simulink model "Task_No4"  (R2023b)
settings: Solver=ode5  StartTime=0.0  StopTime=3600*24*7  FixedStep=1  RelTol=1e-3
InitFcn:
  | PARAMETERS;
StartFcn:
  | PARAMETERS;
values from neighbouring files (symbols this model uses):
  Conv_C_to_K = 273.15    [PARAMETERS.m]
  P_AREA_WALL = sqrt(P_AREA_BDR)*P_RM_HEIGHT-P_AREA_WIN    [PARAMETERS.m]
  P_AREA_WIN = 1.82    [PARAMETERS.m]
  P_CP_AIR = 1012    [PARAMETERS.m]
  P_EM_GLASS = 0.94    [PARAMETERS.m]
  P_EM_WALL = 0.94    [PARAMETERS.m]
  P_HEATER_AIR_FLOW = 1    [PARAMETERS.m]
  R_WALL = 1/(U_WALL*P_AREA_WALL)    [PARAMETERS.m]
  R_WINDOW = 1/(U_WINDOW*P_AREA_WIN)    (= 0.18315018315)    [PARAMETERS.m]
  T_HEATER = 50    [PARAMETERS.m]
  T_INIT_BDR = 18    [PARAMETERS.m]
  T_INIT_OUT = 2.9    [PARAMETERS.m]
undefined symbols (not defined in the file or in its folder): TBL_TEMP
libraries: fl_lib x21, nesl_utility x8, slpidlib x1
settings Model: Creator=Selim  LastModifiedBy=Selim

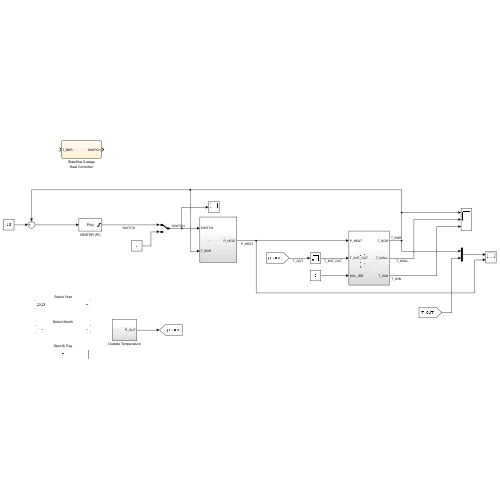
[thumbnail: Simulink's stored preview of the top-level diagram]
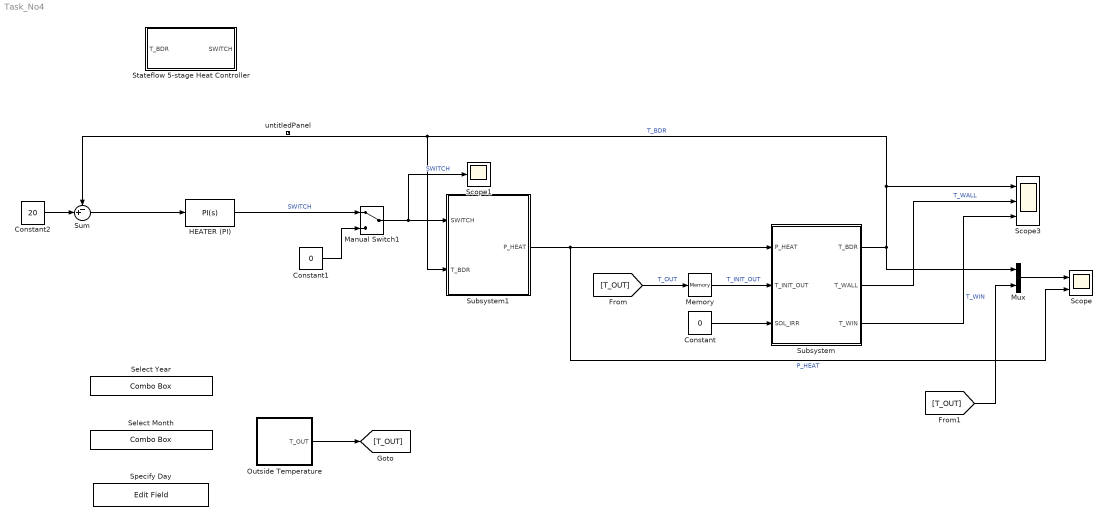
== system Task_No4 ==
  Constant : Constant  Value=0
  Constant1 : Constant  Value=0
  Constant2 : Constant  Value=20
  HEATER (PI) : slpidlib/PID Controller  Controller=PI  Form=Parallel  TimeDomain=Continuous-time  UseExternalTs=off  SampleTime=-1  IntegratorMethod=Forward Euler  FilterMethod=Forward Euler  ControllerParametersSource=internal  P=0.143081964564318  I=0.00336579194559755  UseKiTs=off  D=39.5738922859411  N=3204.37920267902  UseFilter=on  TunerSelectOption=Transfer Function Based (PID Tuner App)  InitialConditionSource=internal  InitialConditionForIntegrator=0  InitialConditionForFilter=0  DifferentiatorICPrevScaledInput=0  ExternalReset=none  TrackingMode=off  Kt=1  LimitOutput=on  SatLimitsSource=internal  UpperSaturationLimit=1  LowerSaturationLimit=0  LinearizeAsGain=on  AntiWindupMode=clamping  Kb=1  LimitIntegrator=off  UpperIntegratorSaturationLimit=inf  LowerIntegratorSaturationLimit=-inf  POutMin=[]  POutMax=[]  IOutMin=[]  IOutMax=[]  DOutMin=[]  DOutMax=[]  NOutMin=[]  NOutMax=[]  SumOutMin=[]  SumOutMax=[]  SaturationOutMin=[]  SaturationOutMax=[]  PParamMin=[]  PParamMax=[]  IParamMin=[]  IParamMax=[]  DParamMin=[]  DParamMax=[]  NParamMin=[]  NParamMax=[]  KbParamMin=[]  KbParamMax=[]  KtParamMin=[]  KtParamMax=[]  KbOutMin=[]  KbOutMax=[]  KtOutMin=[]  KtOutMax=[]  IntegratorOutMin=[]  IntegratorOutMax=[]  FilterOutMin=[]  FilterOutMax=[]  SumI1OutMin=[]  SumI1OutMax=[]  SumI2OutMin=[]  SumI2OutMax=[]  SumI3OutMin=[]  SumI3OutMax=[]  SumI4OutMin=[]  SumI4OutMax=[]  SumDOutMin=[]  SumDOutMax=[]  DifferentiatorOutMin=[]  DifferentiatorOutMax=[]  FilterDiffOutCoefMin=[]  FilterDiffOutCoefMax=[]  ReciprocalOutMin=[]  ReciprocalOutMax=[]  SumDenOutMin=[]  SumDenOutMax=[]  SumNumOutMin=[]  SumNumOutMax=[]  DivideOutMin=[]  DivideOutMax=[]  UdiffTsProdOutMin=[]  UdiffTsProdOutMax=[]  NTsProdOutMin=[]  NTsProdOutMax=[]  UintegralTsProdOutMin=[]  UintegralTsProdOutMax=[]  UngainTsProdOutMin=[]  UngainTsProdOutMax=[]  ClampingZeroOutDataTypeStr=Inherit: Inherit via back propagation  ClampingZeroOutMin=[]  ClampingZeroOutMax=[]  FilterDenConstantOutDataTypeStr=Inherit: Inherit via back propagation  FilterDenConstantOutMin=[]  FilterDenConstantOutMax=[]  PCopyOutDataTypeStr=Inherit: Inherit via back propagation  PCopyOutMin=[]  PCopyOutMax=[]  NCopyOutDataTypeStr=Inherit: Inherit via back propagation  NCopyOutMin=[]  NCopyOutMax=[]  IntegratorContinuousStateAttributes=''  IntegratorStateMustResolveToSignalObject=off  IntegratorRTWStateStorageClass=Auto  FilterContinuousStateAttributes=''  FilterStateMustResolveToSignalObject=off  FilterRTWStateStorageClass=Auto  ParallelPVariant=InternalParameters  IdealPVariant=Disabled  IVariant=InternalParameters  DVariant=Disabled  IntegratorVariant=Continuous  SatVariant=Enabled  AWVariant=ContClampingParallel  PCopyVariant=Disabled  TRVariant=Disabled  FdbkBlocksVariant=Forward  IdealPFdbkVariant=Disabled  SatFdbkVariant=Disabled  DerivativeFilterVariant=Disabled  NVariant=Disabled  NCopyVariant=Disabled_SignalSpec  FilterICVariant=Disabled  IntegratorICVariant=InternalICs  ExternalResetVariant=Disabled  TRSumVariant=Passthrough  SumFdbkVariant=Disabled  SumVariant=Sum_PI  TsampFilterVariant=InternalTs  TsampNgainVariant=Passthrough  TsampIntegralVariant=Disabled_SignalSpec  ExternalSaturationOutDataTypeStr=Inherit: Same as second input
  Manual Switch1 : ManualSwitch
  Memory : Memory  InitialCondition=T_INIT_OUT
  Mux : Mux  Inputs=2
  Outside Temperature : Subsystem
  Scope : Scope  NumInputPorts=2
  Scope1 : Scope
  Scope3 : Scope  NumInputPorts=3
  Select Month : ComboBox  LabelPosition=Hide  SelectedLabel=July
      settings: Values={{'January', 'February', 'March', 'April', 'May', 'June', 'July', 'August', 'September', 'Oktober', 'November', 'December'}, [1 2 3 4 5 6 7 8 9 10 11 12]}
  Select Year : ComboBox  LabelPosition=Hide  SelectedLabel=2023
      settings: Values={{'2022', '2023'}, [2022 2023]}
  Specify Day : EditField  LabelPosition=Hide  ShowInitialText=on  Alignment=Center
  Stateflow 5-stage Heat Controller : Stateflow chart  TreatAsAtomicUnit=on
  Subsystem : Subsystem
  Subsystem1 : Subsystem
  Sum : Sum  Inputs=-+|
  untitledPanel : Subsystem  Tag=HiddenForWebPanel  IsWebBlockPanel=on
  wires:
  Memory/1 -> Subsystem/2(T_INIT_OUT)  "T_INIT_OUT"
  Subsystem/1(T_BDR) -> Sum/1, Subsystem1/2(T_BDR), Scope3/1, Mux/1  "T_BDR"
  Manual Switch1/1 -> Subsystem1/1(SWITCH), Scope1/1  "SWITCH"
  Subsystem1/1(P_HEAT) -> Subsystem/1(P_HEAT), Scope/2  "P_HEAT"
  [T_OUT] -> Memory/1  "T_OUT"
  [T_OUT] -> Mux/2
  Mux/1 -> Scope/1
  Constant/1 -> Subsystem/3(SOL_IRR)
  HEATER (PI)/1 -> Manual Switch1/1  "SWITCH"
  Constant1/1 -> Manual Switch1/2
  Subsystem/2(T_WALL) -> Scope3/2  "T_WALL"
  Subsystem/3(T_WIN) -> Scope3/3  "T_WIN"
  Outside Temperature/1(T_OUT) -> [T_OUT]
  Sum/1 -> HEATER (PI)/1
  Constant2/1 -> Sum/2

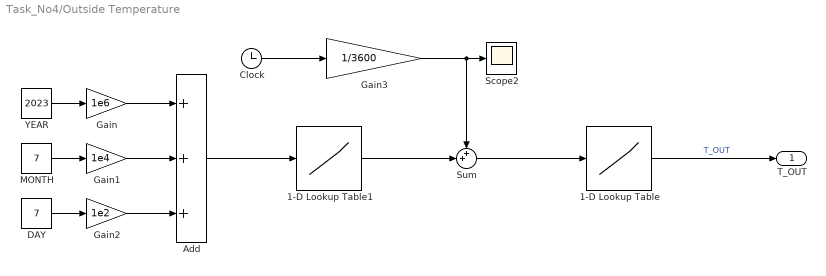
== system Task_No4/Outside Temperature ==
  1-D Lookup Table : Lookup_n-D  NumberOfTableDimensions=1  BreakpointsForDimension1=TBL_TEMP.DATE_sec  Table=TBL_TEMP.T_C  InternalRulePriority=Speed  RndMeth=Simplest
  1-D Lookup Table1 : Lookup_n-D  NumberOfTableDimensions=1  BreakpointsForDimension1=TBL_TEMP.DATE_yyyymmddhh  Table=TBL_TEMP.DATE_sec  InternalRulePriority=Speed  RndMeth=Simplest
  Add : Sum  Inputs=+++
  Clock : Clock
  DAY : Constant  Value=7
  Gain : Gain  Gain=1e6
  Gain1 : Gain  Gain=1e4
  Gain2 : Gain  Gain=1e2
  Gain3 : Gain  Gain=1/3600
  MONTH : Constant  Value=7
  Scope2 : Scope
  Sum : Sum  Inputs=++|
  YEAR : Constant  Value=2023
  T_OUT : Outport
  wires:
  Gain1/1 -> Add/2
  MONTH/1 -> Gain1/1
  Clock/1 -> Gain3/1
  1-D Lookup Table1/1 -> Sum/2
  Add/1 -> 1-D Lookup Table1/1
  YEAR/1 -> Gain/1
  Gain/1 -> Add/1
  Gain3/1 -> Scope2/1, Sum/1
  Sum/1 -> 1-D Lookup Table/1
  Gain2/1 -> Add/3
  DAY/1 -> Gain2/1
  1-D Lookup Table/1 -> T_OUT/1  "T_OUT"

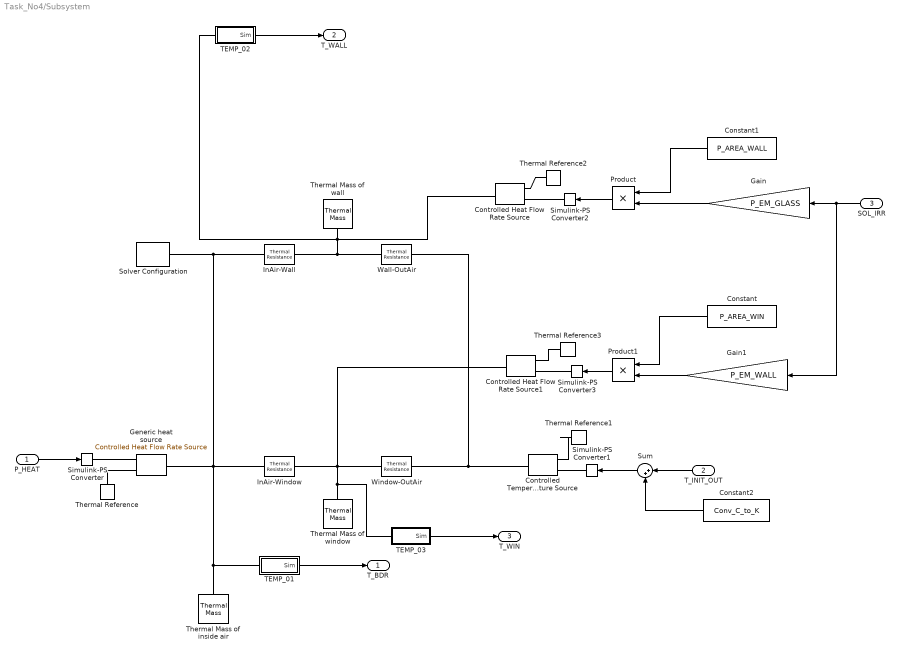
== system Task_No4/Subsystem ==
  P_HEAT : Inport
  T_INIT_OUT : Inport  Port=2
  SOL_IRR : Inport  Port=3
  Constant : Constant  Value=P_AREA_WIN
  Constant1 : Constant  Value=P_AREA_WALL
  Constant2 : Constant  Value=Conv_C_to_K
  Controlled Temperature Source : fl_lib/Thermal/Thermal Sources/Controlled Temperature Source
  Controlled Heat Flow Rate Source : fl_lib/Thermal/Thermal Sources/Controlled Heat Flow Rate Source
  Controlled Heat Flow Rate Source1 : fl_lib/Thermal/Thermal Sources/Controlled Heat Flow Rate Source
  Gain : Gain  Gain=P_EM_GLASS
  Gain1 : Gain  Gain=P_EM_WALL
  Generic heat source : fl_lib/Thermal/Thermal Sources/Controlled Heat Flow Rate Source
  InAir-Wall : fl_lib/Thermal/Thermal Elements/Thermal Resistance  resistance=R_WALL/2 K/W  T_specify=off  T_priority=None  T=0 K  T_nominal_specify=off  T_nominal_unit=K  T_nominal_value=1  Q_specify=off  Q_priority=None  Q=0 W  Q_nominal_specify=off  Q_nominal_unit=W  Q_nominal_value=1
  InAir-Window : fl_lib/Thermal/Thermal Elements/Thermal Resistance  resistance=R_WINDOW/2 K/W  T_specify=off  T_priority=None  T=0 K  T_nominal_specify=off  T_nominal_unit=K  T_nominal_value=1  Q_specify=off  Q_priority=None  Q=0 W  Q_nominal_specify=off  Q_nominal_unit=W  Q_nominal_value=1
  Product : Product
  Product1 : Product
  Simulink-PS Converter{,1..3} (4 alike) : nesl_utility/Simulink-PS Converter  PhysicalDomain=network_engine_domain  SubClassName=ps_input  LeftPortType=input  RightPortType=output  PseudoPeriodic=off  Frequencies=[]  NoiseDistribution=none  NoiseParameters=[]  Unit=1  AffineConversion=off  FilteringAndDerivatives=provide  SimscapeFilterOrder=1  InputFilterTimeConstant=0.001  UdotUserProvided=0
  Solver Configuration : nesl_utility/Solver Configuration  PhysicalDomain=network_engine_domain  SubClassName=solver  LeftPortType=input  RightPortType=generic  Tones=[]  Harmonics=[]  SimulateNoise=off  Profile=off  UseLocalSampling=off  EnableSwitchedLinearOptims=on  FrequencyDomain=off  UseCCode=off  RelTol=0.001  AbsTol=0.001  MinStep=1e-09  ToWorkspace=off  RevertToSquareIcSolve=off  NumHomotopyIterations=100  PhasorMode=off  PhasorModeNumHarmonics=1  ConsistencySolver=NEWTON_XTOL_AFTER_FTOL  IndexReductionMethod=DerivativeReplacement  DoDC=off  ResidualTolerance=1e-09  ConsistencyTolSource=GLOBAL  ConsistencyAbsTol=0.001  ConsistencyRelTol=0.001  ConsistencyTolFactor=0.001  UseLocalSolver=off  LocalSolverChoice=NE_BACKWARD_EULER_ADVANCER  ResolveIndetEquations=on  FunctionEvalNumThread=1  LocalSolverSampleTime=0.001  DoFixedCost=off  MaxNonlinIter=3  MaxModeIter=2  ComputeImpulses=off  ImpulseIterations=2  LinearAlgebra=auto  LinearAlgebraNumThread=0  EquationFormulation=NE_TIME_EF  DelaysMemoryBudget=1024  AutomaticFiltering=on  FilteringTimeConstant=0.001  PartitionStorageMethod=AS_NEEDED  PartitionMemoryBudget=1024  PartitionMethod=ROBUST  MultibodyUseLocalSolver=off  MultibodyLocalSolverChoice=ODE1  MultibodyLocalSolverSampleTime=0.001
  Sum : Sum  Inputs=|++
  TEMP_01 : Subsystem
  TEMP_02 : Subsystem
  TEMP_03 : Subsystem
  Thermal Mass of inside air : fl_lib/Thermal/Thermal Elements/Thermal Mass  mass_type=foundation.enum.constant_variable.constant  mass=P_M_AIR kg  sp_heat=P_CP_AIR J/(K*kg)  mass_min=1e-6 kg  num_ports=foundation.enum.numPorts2.one  m_specify=off  m_priority=High  m=1 kg  m_nominal_specify=off  m_nominal_unit=kg  m_nominal_value=1  T_specify=on  T_priority=High  T=T_INIT_BDR degC  T_nominal_specify=off  T_nominal_unit=K  T_nominal_value=1  Q_specify=off  Q_priority=None  Q=0 W  Q_nominal_specify=off  Q_nominal_unit=W  Q_nominal_value=1
  Thermal Mass of wall : fl_lib/Thermal/Thermal Elements/Thermal Mass  mass_type=foundation.enum.constant_variable.constant  mass=P_M_WALL kg  sp_heat=P_CP_WALL J/(K*kg)  mass_min=1e-6 kg  num_ports=foundation.enum.numPorts2.one  m_specify=off  m_priority=High  m=1 kg  m_nominal_specify=off  m_nominal_unit=kg  m_nominal_value=1  T_specify=on  T_priority=High  T=T_INIT_BDR degC  T_nominal_specify=off  T_nominal_unit=K  T_nominal_value=1  Q_specify=off  Q_priority=None  Q=0 W  Q_nominal_specify=off  Q_nominal_unit=W  Q_nominal_value=1
  Thermal Mass of window : fl_lib/Thermal/Thermal Elements/Thermal Mass  mass_type=foundation.enum.constant_variable.constant  mass=P_M_WINDOW kg  sp_heat=P_CP_GLASS J/(K*kg)  mass_min=1e-6 kg  num_ports=foundation.enum.numPorts2.one  m_specify=off  m_priority=High  m=1 kg  m_nominal_specify=off  m_nominal_unit=kg  m_nominal_value=1  T_specify=on  T_priority=High  T=T_INIT_BDR degC  T_nominal_specify=off  T_nominal_unit=K  T_nominal_value=1  Q_specify=off  Q_priority=None  Q=0 W  Q_nominal_specify=off  Q_nominal_unit=W  Q_nominal_value=1
  Thermal Reference{,1..3} (4 alike) : fl_lib/Thermal/Thermal Elements/Thermal Reference
  Wall-OutAir : fl_lib/Thermal/Thermal Elements/Thermal Resistance  resistance=R_WINDOW/2 K/W  T_specify=off  T_priority=None  T=0 K  T_nominal_specify=off  T_nominal_unit=K  T_nominal_value=1  Q_specify=off  Q_priority=None  Q=0 W  Q_nominal_specify=off  Q_nominal_unit=W  Q_nominal_value=1
  Window-OutAir : fl_lib/Thermal/Thermal Elements/Thermal Resistance  resistance=R_WINDOW/2 K/W  T_specify=off  T_priority=None  T=0 K  T_nominal_specify=off  T_nominal_unit=K  T_nominal_value=1  Q_specify=off  Q_priority=None  Q=0 W  Q_nominal_specify=off  Q_nominal_unit=W  Q_nominal_value=1
  T_BDR : Outport
  T_WALL : Outport  Port=2
  T_WIN : Outport  Port=3
  wires:
  Constant2/1 -> Sum/2
  Sum/1 -> Simulink-PS Converter1/1
  TEMP_01/1(Sim) -> T_BDR/1
  P_HEAT/1 -> Simulink-PS Converter/1
  T_INIT_OUT/1 -> Sum/1
  SOL_IRR/1 -> Gain1/1, Gain/1
  Gain/1 -> Product/2
  Constant1/1 -> Product/1
  Product/1 -> Simulink-PS Converter2/1
  TEMP_02/1(Sim) -> T_WALL/1
  TEMP_03/1(Sim) -> T_WIN/1
  Gain1/1 -> Product1/2
  Constant/1 -> Product1/1
  Product1/1 -> Simulink-PS Converter3/1
  connections:
  Thermal Reference/LConn1 -- Generic heat source/RConn2
  Controlled Temperature Source/LConn1 -- Wall-OutAir/RConn1 -- Window-OutAir/RConn1
  Generic heat source/LConn1 -- Solver Configuration/RConn1 -- InAir-Wall/LConn1 -- InAir-Window/LConn1 -- Thermal Mass of inside air/LConn1 -- TEMP_01/LConn1
  Thermal Reference1/LConn1 -- Controlled Temperature Source/RConn2
  Simulink-PS Converter/RConn1 -- Generic heat source/RConn1
  Simulink-PS Converter1/RConn1 -- Controlled Temperature Source/RConn1
  Simulink-PS Converter2/RConn1 -- Controlled Heat Flow Rate Source/RConn1
  Thermal Reference2/LConn1 -- Controlled Heat Flow Rate Source/RConn2
  Window-OutAir/LConn1 -- Controlled Heat Flow Rate Source1/LConn1 -- TEMP_03/LConn1 -- Thermal Mass of window/LConn1 -- InAir-Window/RConn1
  InAir-Wall/RConn1 -- Controlled Heat Flow Rate Source/LConn1 -- TEMP_02/LConn1 -- Thermal Mass of wall/LConn1 -- Wall-OutAir/LConn1
  Controlled Heat Flow Rate Source1/RConn1 -- Simulink-PS Converter3/RConn1
  Thermal Reference3/LConn1 -- Controlled Heat Flow Rate Source1/RConn2

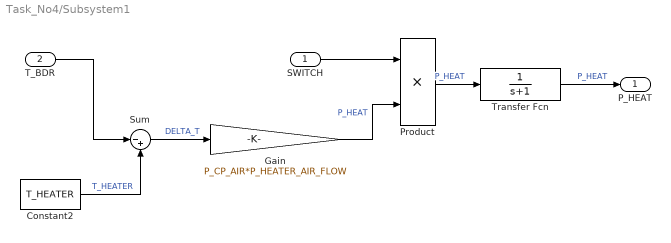
== system Task_No4/Subsystem1 ==
  SWITCH : Inport
  T_BDR : Inport  Port=2
  Constant2 : Constant  Value=T_HEATER
  Gain : Gain  Gain=P_CP_AIR*P_HEATER_AIR_FLOW
  Product : Product
  Sum : Sum  Inputs=|-+
  Transfer Fcn : TransferFcn  Denominator=[1 1]
  P_HEAT : Outport
  wires:
  Sum/1 -> Gain/1  "DELTA_T"
  Transfer Fcn/1 -> P_HEAT/1  "P_HEAT"
  Constant2/1 -> Sum/2  "T_HEATER"
  SWITCH/1 -> Product/1
  Gain/1 -> Product/2  "P_HEAT"
  T_BDR/1 -> Sum/1
  Product/1 -> Transfer Fcn/1  "P_HEAT"

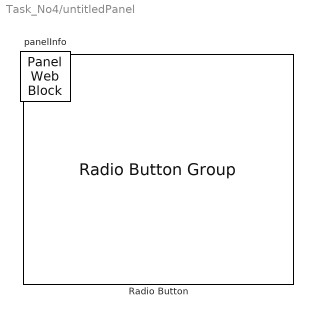
== system Task_No4/untitledPanel ==
  Radio Button : RadioButtonGroup  Tag=HiddenForWebPanel  PanelInfo="{\"addnFilesFolder\":\"\",\"height\":230,\"includeDebugPackages\":false,\"left\":18,\"outputFolder\":\"\",\"panelId\":\"panelId-a10107d6-1e7d-451d-956e-0df6eada92c1\",\"popoutMode\":\"\",\"standaloneTitle\":\"\",\"top\":18,\"type\":\"panelChild\",\"version\":\"2019b\",\"width\":270,\"zIndex\":1500002}"  SelectedLabel=Label3  ButtonGroupName=Group
      settings: Values={{'Label1', 'Label2', 'Label3'}, [0 1 2]}
  panelInfo : PanelWebBlock  Tag=HiddenForWebPanel  PanelInfo="{\"addnFilesFolder\":\"\",\"compacted\":false,\"height\":270,\"includeDebugPackages\":false,\"isActiveTab\":true,\"left\":296,\"name\":\"Panel\",\"outputFolder\":\"\",\"panelId\":\"panelId-a10107d6-1e7d-451d-956e-0df6eada92c1\",\"popoutData\":{\"height\":334,\"left\":361,\"maximized\":false,\"top\":306,\"width\":324},\"popoutMode\":\"windowHidden\",\"standaloneTitle\":\"\",\"tabIndex\":0,\"tabbedSetId\":\"tabbedSet8433950298\",\"top\":135,\"type\":\"panel\",\"version\":\"2019b\",\"visible\":true,\"width\":310,\"zIndex\":1500002}"

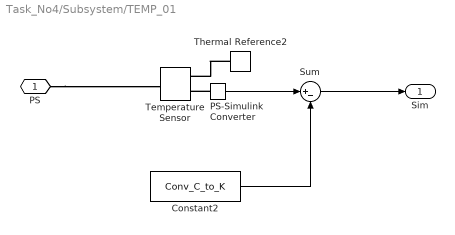
== system Task_No4/Subsystem/TEMP_01 ==
  Constant2 : Constant  Value=Conv_C_to_K
  PS-Simulink Converter : nesl_utility/PS-Simulink Converter  PhysicalDomain=network_engine_domain  SubClassName=ps_output  LeftPortType=input  RightPortType=output  PseudoPeriodic=off  Frequencies=[]  VectorFormat=inherit  Unit=inherit  AffineConversion=off
  Sum : Sum  Inputs=|+-
  Temperature Sensor : fl_lib/Thermal/Thermal Sensors/Temperature Sensor  temperature_measure=foundation.enum.MeasurementReference.difference
  Thermal Reference2 : fl_lib/Thermal/Thermal Elements/Thermal Reference
  PS : PMIOPort  Side=Left
  Sim : Outport
  wires:
  Sum/1 -> Sim/1
  PS-Simulink Converter/1 -> Sum/1
  Constant2/1 -> Sum/2
  connections:
  Thermal Reference2/LConn1 -- Temperature Sensor/RConn1
  PS-Simulink Converter/LConn1 -- Temperature Sensor/RConn2
  PS/RConn1 -- Temperature Sensor/LConn1

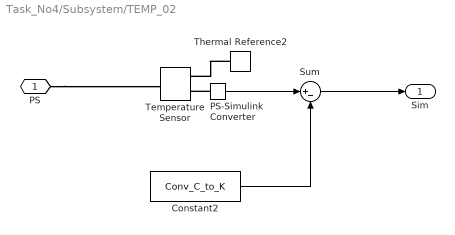
== system Task_No4/Subsystem/TEMP_02 ==
  Constant2 : Constant  Value=Conv_C_to_K
  PS-Simulink Converter : nesl_utility/PS-Simulink Converter  PhysicalDomain=network_engine_domain  SubClassName=ps_output  LeftPortType=input  RightPortType=output  PseudoPeriodic=off  Frequencies=[]  VectorFormat=inherit  Unit=inherit  AffineConversion=off
  Sum : Sum  Inputs=|+-
  Temperature Sensor : fl_lib/Thermal/Thermal Sensors/Temperature Sensor  temperature_measure=foundation.enum.MeasurementReference.difference
  Thermal Reference2 : fl_lib/Thermal/Thermal Elements/Thermal Reference
  PS : PMIOPort  Side=Left
  Sim : Outport
  wires:
  Sum/1 -> Sim/1
  PS-Simulink Converter/1 -> Sum/1
  Constant2/1 -> Sum/2
  connections:
  Thermal Reference2/LConn1 -- Temperature Sensor/RConn1
  PS-Simulink Converter/LConn1 -- Temperature Sensor/RConn2
  PS/RConn1 -- Temperature Sensor/LConn1

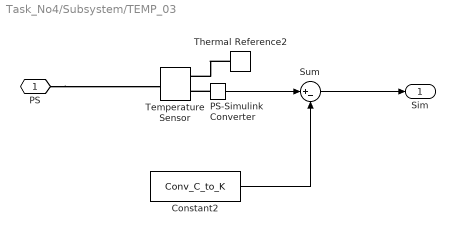
== system Task_No4/Subsystem/TEMP_03 ==
  Constant2 : Constant  Value=Conv_C_to_K
  PS-Simulink Converter : nesl_utility/PS-Simulink Converter  PhysicalDomain=network_engine_domain  SubClassName=ps_output  LeftPortType=input  RightPortType=output  PseudoPeriodic=off  Frequencies=[]  VectorFormat=inherit  Unit=inherit  AffineConversion=off
  Sum : Sum  Inputs=|+-
  Temperature Sensor : fl_lib/Thermal/Thermal Sensors/Temperature Sensor  temperature_measure=foundation.enum.MeasurementReference.difference
  Thermal Reference2 : fl_lib/Thermal/Thermal Elements/Thermal Reference
  PS : PMIOPort  Side=Left
  Sim : Outport
  wires:
  Sum/1 -> Sim/1
  PS-Simulink Converter/1 -> Sum/1
  Constant2/1 -> Sum/2
  connections:
  Thermal Reference2/LConn1 -- Temperature Sensor/RConn1
  PS-Simulink Converter/LConn1 -- Temperature Sensor/RConn2
  PS/RConn1 -- Temperature Sensor/LConn1

== stateflow chart Task_No4/Stateflow 5-stage Heat Controller ==
  state Off
    entry:
    SWITCH = 0;
  state Low
    entry:
    SWITCH = 0.25;
  state Medium
    entry:
    SWITCH = 0.5;
  state High
    entry:
    SWITCH = 0.75;
  state Full
    entry:
    SWITCH = 1;
  (default) -> Off
  Low -> Medium [order 2] : [T_BDR<20]
  High -> Full [order 2] : [T_BDR<18]
  Off -> Low : [T_BDR<21]
  Medium -> High [order 2] : [T_BDR<19]
  Low -> Off [order 1] : [T_BDR>=22]
  Medium -> Low [order 1] : [T_BDR>=21]
  High -> Medium [order 1] : [T_BDR>=20]
  Full -> High : [T_BDR>=20]
  data: T_BDR input; SWITCH output
